simulink model "PID_control"  (R2017b)
settings: Solver=ode4  StartTime=0.0  StopTime=10  FixedStep=0.01  RelTol=1e-3
undefined symbols (not defined in the file or in its folder): K_muS, Kd, Ki, Kp, muS
settings Model: Creator=84935  LastModifiedBy=84935
settings RTWCC: GenerateReport=on  LaunchReport=on

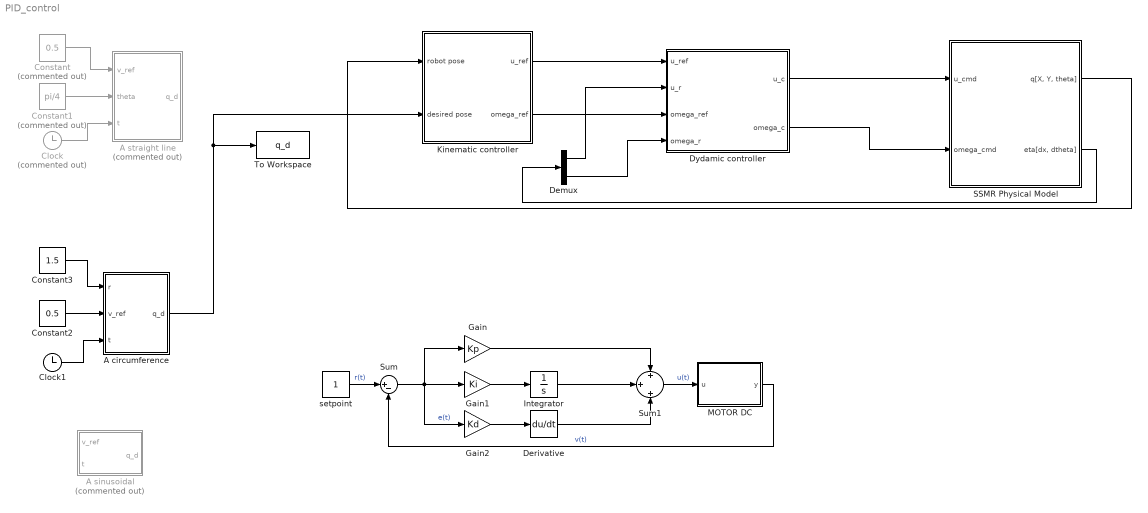
== system PID_control ==
  A circumference : MATLAB Function  TreatAsAtomicUnit=on
  A sinusoidal : MATLAB Function  Commented=on  TreatAsAtomicUnit=on
  A straight line : MATLAB Function  Commented=on  TreatAsAtomicUnit=on
  Clock : Clock  Commented=on
  Clock1 : Clock
  Constant : Constant  Commented=on  Value=0.5
  Constant1 : Constant  Commented=on  Value=pi/4
  Constant2 : Constant  Value=0.5
  Constant3 : Constant  Value=1.5
  Demux : Demux  Outputs=2
  Derivative : Derivative
  Dydamic controller : Subsystem  mask{FF_u=0, FF_omega=0, Kp_u=0, Ki_u=0, Kp_omega=0, Ki_omega=0}
  Gain : Gain  Gain=Kp
  Gain1 : Gain  Gain=Ki
  Gain2 : Gain  Gain=Kd
  Integrator : Integrator
  Kinematic controller : Subsystem  mask{Kp_rho=0, Ki_rho=0, Kp_XTE=0, Ki_XTE=0, Kp_theta=0, Ki_theta=0}
      mask prompts: Kp_rho "Kp rho"; Ki_rho "Ki rho"; Kp_XTE "Kp XTE"; Ki_XTE "Ki XTE"; Kp_theta "Kp theta"; Ki_theta "Ki theta"
  MOTOR DC : MATLAB Function  TreatAsAtomicUnit=on
  SSMR Physical Model : Subsystem  mask{K_w=1, r=0.0625, m=1, g=9.81, K_ux=1, W=0.29821, J_z=1, K_theta=1, vx_max=1, w_max=1, delay_u=1, delay_w=1}
      mask prompts: K_w "K_w unknow parameter"; r "radius wheel (m)"; m "vehicle mass (kg)"; g "gravitational acceleration (m/s2)"; K_ux "K_ux unknow parameter"; W "vehicle width (m)"; J_z "J_z = WI/4"; K_theta "K_theta unknow parameter"; vx_max "vx_max (m/s)"; w_max "w_max (rad/s)"; delay_u "delay_u unknow parameter (s)"; delay_w "delay_w unknow parameter (s)"
  Sum : Sum  Inputs=|+-
  Sum1 : Sum  Inputs=+|+|+
  To Workspace : ToWorkspace  VariableName=q_d  SaveFormat=Structure  SampleTime=-1
  setpoint : Constant
  wires:
  Dydamic controller/1(u_c) -> SSMR Physical Model/1(u_cmd)
  Dydamic controller/2(omega_c) -> SSMR Physical Model/2("omega_cmd ")
  SSMR Physical Model/2("eta[dx, dtheta]") -> Demux/1
  Kinematic controller/1(u_ref) -> Dydamic controller/1(u_ref)
  Kinematic controller/2(omega_ref) -> Dydamic controller/3(omega_ref)
  Demux/1 -> Dydamic controller/2(u_r)
  Demux/2 -> Dydamic controller/4(omega_r)
  Constant/1 -> A straight line/1(v_ref)
  SSMR Physical Model/1("q[X, Y, theta] ") -> Kinematic controller/1(robot pose)
  Clock/1 -> A straight line/3(t)
  Constant1/1 -> A straight line/2(theta)
  Constant2/1 -> A circumference/2(v_ref)
  Constant3/1 -> A circumference/1(r)
  Clock1/1 -> A circumference/3(t)
  A circumference/1(q_d) -> Kinematic controller/2(desired pose), To Workspace/1
  Gain1/1 -> Integrator/1
  Gain2/1 -> Derivative/1
  Sum/1 -> Gain2/1, Gain/1, Gain1/1  "e(t)"
  Gain/1 -> Sum1/1
  Integrator/1 -> Sum1/2
  Derivative/1 -> Sum1/3
  Sum1/1 -> MOTOR DC/1(u)  "u(t)"
  MOTOR DC/1(y) -> Sum/2  "v(t)"
  setpoint/1 -> Sum/1  "r(t)"

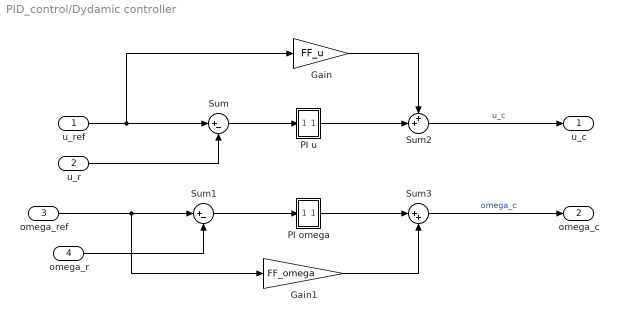
== system PID_control/Dydamic controller ==
  u_ref : Inport
  u_r : Inport  Port=2
  omega_ref : Inport  Port=3
  omega_r : Inport  Port=4
  Gain : Gain  Gain=FF_u
  Gain1 : Gain  Gain=FF_omega
  PI omega : Subsystem
  PI u : Subsystem
  Sum : Sum  Inputs=|+-
  Sum1 : Sum  Inputs=|+-
  Sum2 : Sum  Inputs=++|
  Sum3 : Sum  Inputs=|++
  u_c : Outport
  omega_c : Outport  Port=2
  wires:
  Gain1/1 -> Sum3/2
  PI omega/1(u) -> Sum3/1
  PI u/1(u) -> Sum2/2
  u_r/1 -> Sum/2
  Gain/1 -> Sum2/1
  Sum/1 -> PI u/1(e)
  Sum3/1 -> omega_c/1  "omega_c"
  omega_ref/1 -> Gain1/1, Sum1/1
  Sum1/1 -> PI omega/1(e)
  u_ref/1 -> Gain/1, Sum/1
  Sum2/1 -> u_c/1  "u_c"
  omega_r/1 -> Sum1/2

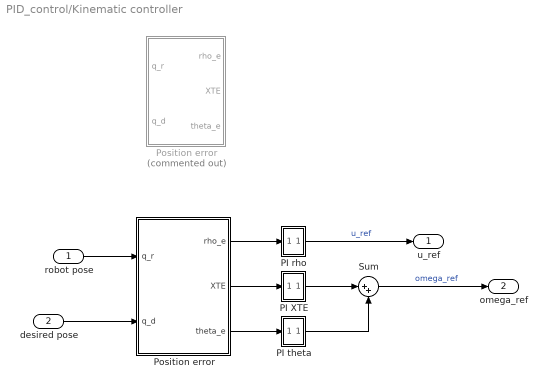
== system PID_control/Kinematic controller ==
  robot pose : Inport
  desired pose : Inport  Port=2
  PI XTE : Subsystem
  PI rho : Subsystem
  PI theta : Subsystem
  Position error : MATLAB Function  TreatAsAtomicUnit=on
  "Position error " : Subsystem  Commented=on
  Sum : Sum  Inputs=|++
  u_ref : Outport
  omega_ref : Outport  Port=2
  wires:
  robot pose/1 -> Position error/1(q_r)
  PI XTE/1(u) -> Sum/1
  PI theta/1(u) -> Sum/2
  Sum/1 -> omega_ref/1  "omega_ref"
  Position error/2(XTE) -> PI XTE/1(e)
  Position error/3(theta_e) -> PI theta/1(e)
  PI rho/1(u) -> u_ref/1  "u_ref"
  Position error/1(rho_e) -> PI rho/1(e)
  desired pose/1 -> Position error/2(q_d)

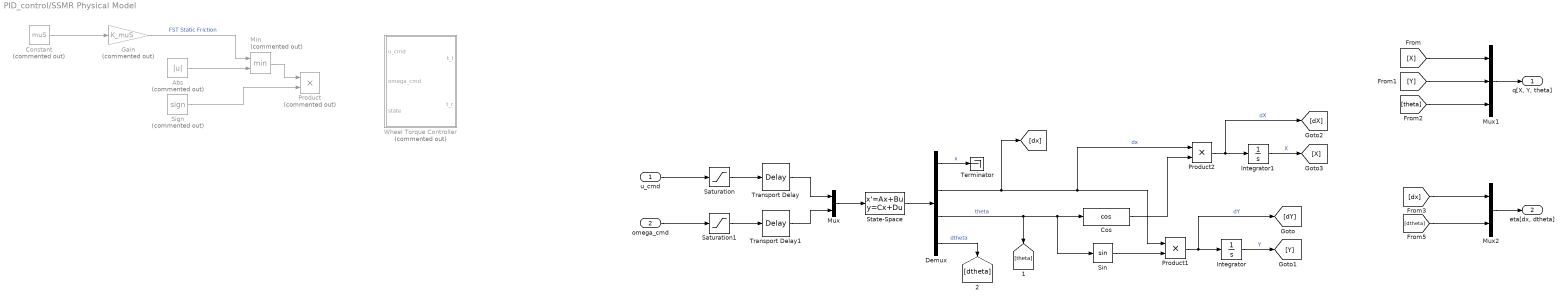
== system PID_control/SSMR Physical Model ==
  u_cmd : Inport
  "omega_cmd " : Inport  Port=2
  Abs : Abs  Commented=on
  Constant : Constant  Commented=on  Value=muS
  Cos : Trigonometry  Operator=cos
  Demux : Demux
  Gain : Gain  Commented=on  Gain=K_muS
  Integrator : Integrator
  Integrator1 : Integrator
  Min : MinMax  Commented=on  Inputs=2
  Mux : Mux  Inputs=2
  Mux1 : Mux  Inputs=3
  Mux2 : Mux  Inputs=2
  Product : Product  Commented=on
  Product1 : Product
  Product2 : Product
  Saturation : Saturate  UpperLimit=vx_max  LowerLimit=-vx_max
  Saturation1 : Saturate  UpperLimit=w_max  LowerLimit=-w_max
  Sign : Signum  Commented=on
  Sin : Trigonometry
  State-Space : StateSpace  A=[ 0 1 0 0; 0 (-2*K_w/(r*m)-m*g*K_ux) 0 0; 0 0 0 1; 0 0 0 (-K_w*W*W/(2*r*J_z)-m*g*K_theta*W/(2*J_z))]  B=[0 0; 2*K_w/(r*m) 0; 0 0; 0 K_w*W*W/(2*r*J_z)]  C=[1 0 0 0; 0 1 0 0; 0 0 1 0; 0 0 0 1]  D=[0 0; 0 0; 0 0; 0 0]  InitialCondition=0
  Terminator : Terminator
  Transport Delay : TransportDelay  DelayTime=delay_u
  Transport Delay1 : TransportDelay  DelayTime=delay_w
  Wheel Torque Controller : Subsystem  Commented=on  mask{W=0.29821, r=0.0625, K_w=0, t_max=0}
      mask prompts: W "Width of the vehicle (m)"; r "Wheel radius (m)"; K_w "K_w (unknow parameter)"; t_max "Maximun moment (unknow parameter) (N.m)"
  "q[X, Y, theta] " : Outport
  "eta[dx, dtheta]" : Outport  Port=2
  wires:
  Constant/1 -> Gain/1
  Gain/1 -> Min/1  "FST Static Friction"
  Abs/1 -> Min/2
  Min/1 -> Product/1
  Sign/1 -> Product/2
  u_cmd/1 -> Saturation/1
  "omega_cmd "/1 -> Saturation1/1
  Saturation/1 -> Transport Delay/1
  Saturation1/1 -> Transport Delay1/1
  Transport Delay/1 -> Mux/1
  Transport Delay1/1 -> Mux/2
  Mux/1 -> State-Space/1
  State-Space/1 -> Demux/1
  Demux/1 -> Terminator/1  "x"
  Demux/2 -> Product2/1, Product1/1, [dx]  "dx"
  Demux/4 -> [dtheta]  "dtheta"
  Demux/3 -> [theta], Sin/1, Cos/1  "theta"
  Sin/1 -> Product1/2
  Product1/1 -> [dY], Integrator/1  "dY"
  Integrator/1 -> [Y]  "Y"
  Integrator1/1 -> [X]  "X"
  Cos/1 -> Product2/2
  Product2/1 -> [dX], Integrator1/1  "dX"
  [X] -> Mux1/1
  [Y] -> Mux1/2
  [theta] -> Mux1/3
  Mux1/1 -> "q[X, Y, theta] "/1
  Mux2/1 -> "eta[dx, dtheta]"/1
  [dx] -> Mux2/1
  [dtheta] -> Mux2/2

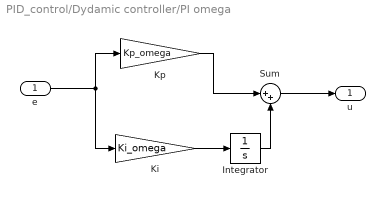
== system PID_control/Dydamic controller/PI omega ==
  e : Inport
  Integrator : Integrator
  Ki : Gain  Gain=Ki_omega
  Kp : Gain  Gain=Kp_omega
  Sum : Sum  Inputs=|++
  u : Outport
  wires:
  Sum/1 -> u/1
  Ki/1 -> Integrator/1
  Integrator/1 -> Sum/2
  Kp/1 -> Sum/1
  e/1 -> Ki/1, Kp/1

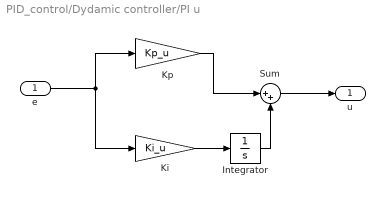
== system PID_control/Dydamic controller/PI u ==
  e : Inport
  Integrator : Integrator
  Ki : Gain  Gain=Ki_u
  Kp : Gain  Gain=Kp_u
  Sum : Sum  Inputs=|++
  u : Outport
  wires:
  Sum/1 -> u/1
  Ki/1 -> Integrator/1
  Integrator/1 -> Sum/2
  Kp/1 -> Sum/1
  e/1 -> Ki/1, Kp/1

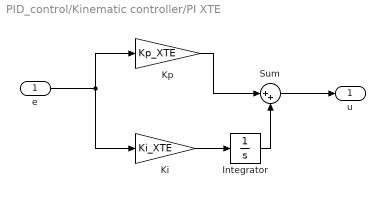
== system PID_control/Kinematic controller/PI XTE ==
  e : Inport
  Integrator : Integrator
  Ki : Gain  Gain=Ki_XTE
  Kp : Gain  Gain=Kp_XTE
  Sum : Sum  Inputs=|++
  u : Outport
  wires:
  Sum/1 -> u/1
  Ki/1 -> Integrator/1
  Integrator/1 -> Sum/2
  Kp/1 -> Sum/1
  e/1 -> Ki/1, Kp/1

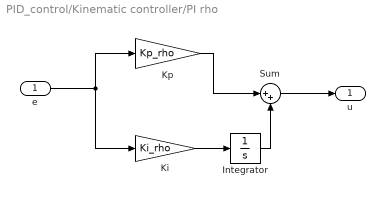
== system PID_control/Kinematic controller/PI rho ==
  e : Inport
  Integrator : Integrator
  Ki : Gain  Gain=Ki_rho
  Kp : Gain  Gain=Kp_rho
  Sum : Sum  Inputs=|++
  u : Outport
  wires:
  Sum/1 -> u/1
  Ki/1 -> Integrator/1
  Integrator/1 -> Sum/2
  Kp/1 -> Sum/1
  e/1 -> Ki/1, Kp/1

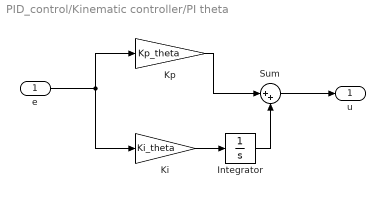
== system PID_control/Kinematic controller/PI theta ==
  e : Inport
  Integrator : Integrator
  Ki : Gain  Gain=Ki_theta
  Kp : Gain  Gain=Kp_theta
  Sum : Sum  Inputs=|++
  u : Outport
  wires:
  Sum/1 -> u/1
  Ki/1 -> Integrator/1
  Integrator/1 -> Sum/2
  Kp/1 -> Sum/1
  e/1 -> Ki/1, Kp/1

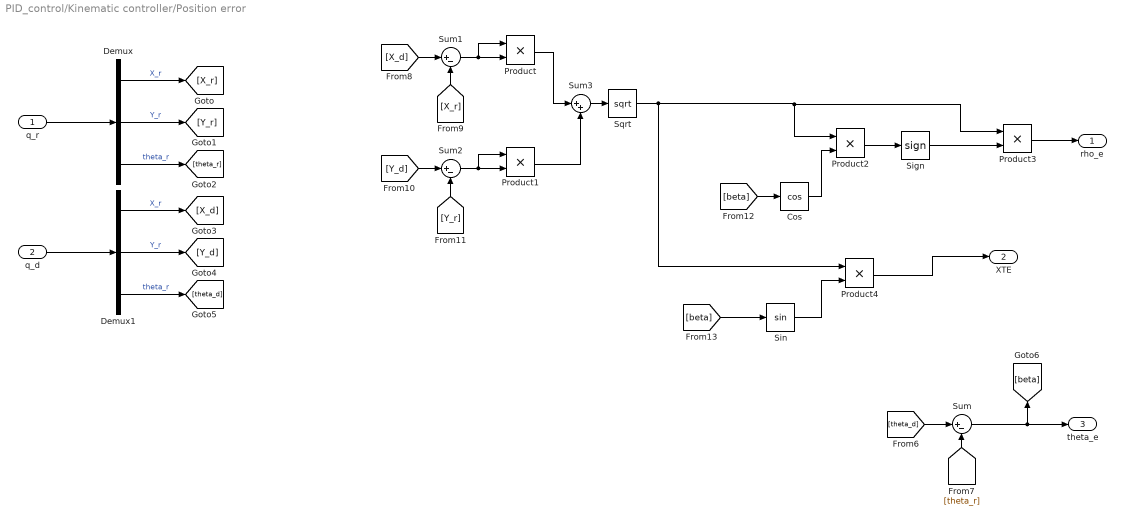
== system PID_control/Kinematic controller/Position error  ==
  q_r : Inport
  q_d : Inport  Port=2
  Cos : Trigonometry  Operator=cos
  Demux : Demux  Outputs=3
  Demux1 : Demux  Outputs=3
  Product{,1..4} (5 alike) : Product
  Sign : Signum
  Sin : Trigonometry
  Sqrt : Sqrt  SaturateOnIntegerOverflow=on
  Sum : Sum  Inputs=|+-
  Sum1 : Sum  Inputs=|+-
  Sum2 : Sum  Inputs=|+-
  Sum3 : Sum  Inputs=|++
  rho_e : Outport
  XTE : Outport  Port=2
  theta_e : Outport  Port=3
  wires:
  q_r/1 -> Demux/1
  q_d/1 -> Demux1/1
  Demux/1 -> [X_r]  "X_r"
  Demux/2 -> [Y_r]  "Y_r"
  Demux/3 -> [theta_r]  "theta_r"
  Demux1/3 -> [theta_d]  "theta_r"
  Demux1/2 -> [Y_d]  "Y_r"
  Demux1/1 -> [X_d]  "X_r"
  Sum/1 -> [beta], theta_e/1
  [theta_d] -> Sum/1
  [theta_r] -> Sum/2
  [X_d] -> Sum1/1
  [X_r] -> Sum1/2
  Sum1/1 -> Product/1, Product/2
  Sum2/1 -> Product1/1, Product1/2
  [Y_d] -> Sum2/1
  [Y_r] -> Sum2/2
  Product/1 -> Sum3/1
  Product1/1 -> Sum3/2
  Sum3/1 -> Sqrt/1
  [beta] -> Cos/1
  Product3/1 -> rho_e/1
  Cos/1 -> Product2/2
  Product2/1 -> Sign/1
  Sign/1 -> Product3/2
  Sqrt/1 -> Product4/1, Product3/1, Product2/1
  Product4/1 -> XTE/1
  [beta] -> Sin/1
  Sin/1 -> Product4/2

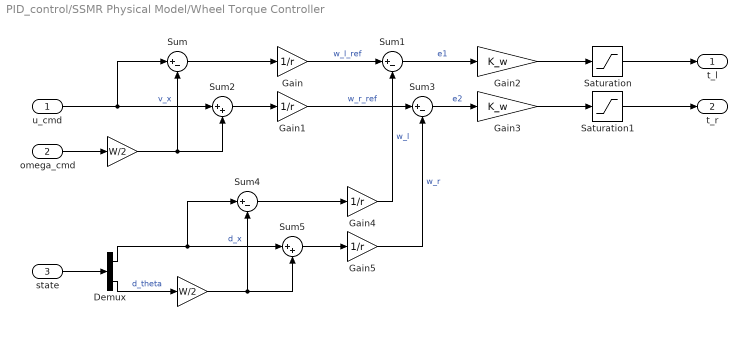
== system PID_control/SSMR Physical Model/Wheel Torque Controller ==
  u_cmd : Inport
  "omega_cmd " : Inport  Port=2
  state : Inport  Port=3
  " " : Gain  Gain=W/2
  " " : Gain  Gain=W/2
  Demux : Demux  Outputs=2
  Gain{,1,4..5} (4 alike) : Gain  Gain=1/r
  Gain2 : Gain  Gain=K_w
  Gain3 : Gain  Gain=K_w
  Saturation : Saturate  UpperLimit=t_max  LowerLimit=-t_max
  Saturation1 : Saturate  UpperLimit=t_max  LowerLimit=-t_max
  Sum{,1,3..4} (4 alike) : Sum  Inputs=|+-
  Sum2 : Sum  Inputs=|++
  Sum5 : Sum  Inputs=|++
  t_l : Outport
  t_r : Outport  Port=2
  wires:
  Gain/1 -> Sum1/1  "w_l_ref"
  Sum2/1 -> Gain1/1
  Gain1/1 -> Sum3/1  "w_r_ref"
  Gain2/1 -> Saturation/1
  Sum5/1 -> Gain5/1
  Demux/1 -> Sum5/1, Sum4/1  "d_x"
  Sum4/1 -> Gain4/1
  Demux/2 -> " "/1  "d_theta"
  " "/1 -> Sum5/2, Sum4/2
  Gain5/1 -> Sum3/2  "w_r"
  Gain4/1 -> Sum1/2  "w_l"
  " "/1 -> Sum2/2, Sum/2
  u_cmd/1 -> Sum2/1, Sum/1  "v_x"
  "omega_cmd "/1 -> " "/1
  Saturation/1 -> t_l/1
  Sum/1 -> Gain/1
  state/1 -> Demux/1
  Sum1/1 -> Gain2/1  "e1"
  Gain3/1 -> Saturation1/1
  Sum3/1 -> Gain3/1  "e2"
  Saturation1/1 -> t_r/1

== matlab function PID_control/A straight line ==
  data: v_ref input; q_d output; theta input; t input
    function q_d      = fcn(v_ref, theta, t)
    % q_d[X, Y, theta]
    q_d = zeros(3, 1);
    q_d(1) = v_ref*t*cos(theta);
    q_d(2) = v_ref*t*sin(theta);
    q_d(3) = theta;

== matlab function PID_control/Kinematic controller/Position error ==
  data: q_r input; rho_e output; q_d input; XTE output; theta_e output
function [rho_e, XTE, theta_e] = fcn(q_r, q_d)
%q_r [X_r, Y_r, theta_r]
%q_d [X_d, Y_d, theta_d]
theta_e = q_d(3) - q_r(3);
distance = sqrt((q_d(1)-q_r(1)).^2+(q_d(2)-q_r(2)).^2);
XTE = distance*sin(theta_e);
rho_e = distance*sign(distance*cos(theta_e));

== matlab function PID_control/A circumference ==
  data: q_d output; r input; v_ref input; t input
function q_d = fcn(r, v_ref, t)
% q_d[X, Y, theta]
  q_d = zeros(3, 1);
  q_d(1)=r*cos(v_ref*t/r);
  q_d(2)=r*sin(v_ref*t/r);
  q_d(3)=pi/2 + v_ref*t/r;

== matlab function PID_control/A sinusoidal ==
  data: v_ref input; q_d output; t input
function  q_d = fcn(v_ref, t)
% q_d[X, Y, theta]
q_d = zeros(3, 1);
if t < 1.5
    q_d(1) = v_ref*t;
    q_d(2) = 0;
    q_d(3)  = 0;
else 
    q_d(1) = v_ref*t;
    q_d(2) = 0.5*sin(0.1*pi*(t-1.5));
    q_d(3) = 0;
end

== matlab function PID_control/MOTOR DC ==
  data: u input; y output
function y = fcn(u)

y = u;
